simulink model "assignment2_2"  (R2016b)
settings: Solver=VariableStepAuto  StartTime=0.0  StopTime=10  RelTol=1e-3
InitFcn:
  | assignment2_1
StartFcn:
  | assignment2_1
values from neighbouring files (symbols this model uses):
  A = [	0, 1, 0, 0; 	-K_lin/J_1, -(K_m*N)^2/(R_m*J_1), K_lin/J_1, 0; 	0, 0, 0, 1; 	K_lin/J_2, 0, -K_lin/J_2, 0]    [assignment2_1.m]    (also in assignment2_3.m)
  B = [	0; 	(N*K_m)/(R_m*J_1); 	0; 	0]    [assignment2_1.m]    (also in assignment2_3.m)
  C = [1, 0, 0, 0 ... (first row only)    [assignment2_1.m]    (also in assignment2_3.m)
  D = [0; 0]    [assignment2_1.m]    (also in assignment2_3.m)
settings Model: Creator=rickardandersson  LastModifiedBy=rickardandersson

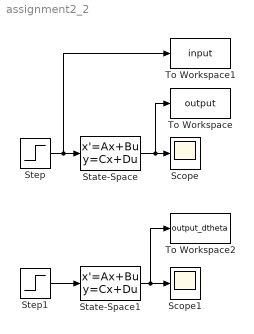
== system assignment2_2 ==
  Scope : Scope
  Scope1 : Scope
  State-Space : StateSpace  A=A  B=B  C=C  D=D  X0=0
  State-Space1 : StateSpace  A=A  B=B  C=[0 1 0 0]  D=[0]  X0=0
  Step : Step  SampleTime=0
  Step1 : Step  SampleTime=0
  To Workspace : ToWorkspace  VariableName=output  SaveFormat=Timeseries  SampleTime=-1
  To Workspace1 : ToWorkspace  VariableName=input  SaveFormat=Timeseries  SampleTime=-1
  To Workspace2 : ToWorkspace  VariableName=output_dtheta  SaveFormat=Timeseries  SampleTime=-1
  wires:
  Step/1 -> To Workspace1/1, State-Space/1
  State-Space/1 -> To Workspace/1, Scope/1
  Step1/1 -> State-Space1/1
  State-Space1/1 -> To Workspace2/1, Scope1/1
